simulink model "TP_MCA_QTP"  (R2025b)
settings: Solver=ode4  StartTime=0.0  StopTime=1000  FixedStep=1e-3  RelTol=1e-3
values from neighbouring files (symbols this model uses):
  A = full(A)    [Parameters.m]
  B = full(B)    [Parameters.m]
  QTP = {}    [Parameters.m]
  uref = sol(3:4)    [Parameters.m]
  xref = [href; sol(1:2)]    [Parameters.m]
undefined symbols (not defined in the file or in its folder): K
settings Model: Creator=yuqi  LastModifiedBy=flo

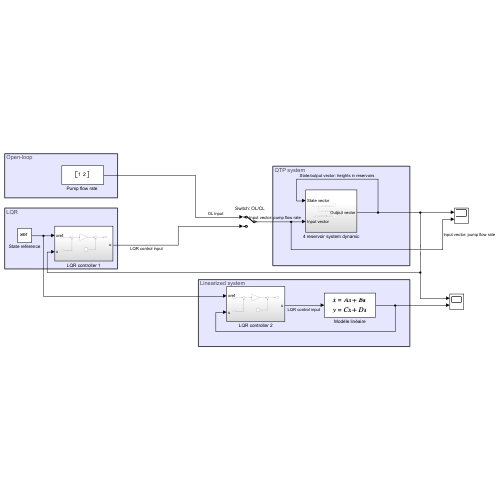
[thumbnail: Simulink's stored preview of the top-level diagram]
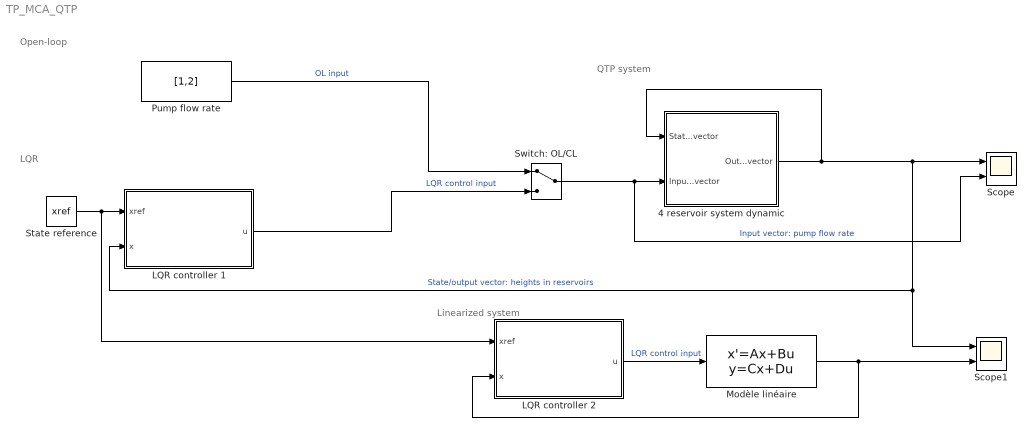
== system TP_MCA_QTP ==
  note: Linearized system
  note: Open-loop
  note: LQR
  note: QTP system
  4 reservoir system dynamic : Subsystem
  LQR controller 1 : Subsystem
  LQR controller 2 : Subsystem
  Modèle linéaire : StateSpace  A=A  B=B  C=eye(4)  D=zeros(4,2)  InitialCondition=QTP.h0
  "Pump flow rate " : Constant  Value=[1,2]
  Scope : Scope  NumInputPorts=2
      settings: ActiveDisplayYMinimum=-0.14202036556311504  ActiveDisplayYMaximum=1.3368369279989929
  Scope1 : Scope  NumInputPorts=2
      settings: ActiveDisplayYMinimum=-0.14887499999999998  ActiveDisplayYMaximum=1.349875
  State reference : Constant  Value=xref
  Switch: OL/CL : ManualSwitch
  wires:
  4 reservoir system dynamic/1(Output vector) -> Scope1/1, LQR controller 1/2(x), Scope/1, 4 reservoir system dynamic/1(State vector)  "State/output vector: heights in reservoirs"
  Switch: OL/CL/1 -> Scope/2, 4 reservoir system dynamic/2(Input vector)  "Input vector: pump flow rate"
  "Pump flow rate "/1 -> Switch: OL/CL/1  "OL input"
  State reference/1 -> LQR controller 2/1(xref), LQR controller 1/1(xref)
  LQR controller 1/1(u) -> Switch: OL/CL/2  "LQR control input"
  Modèle linéaire/1 -> LQR controller 2/2(x), Scope1/2
  LQR controller 2/1(u) -> Modèle linéaire/1  "LQR control input"

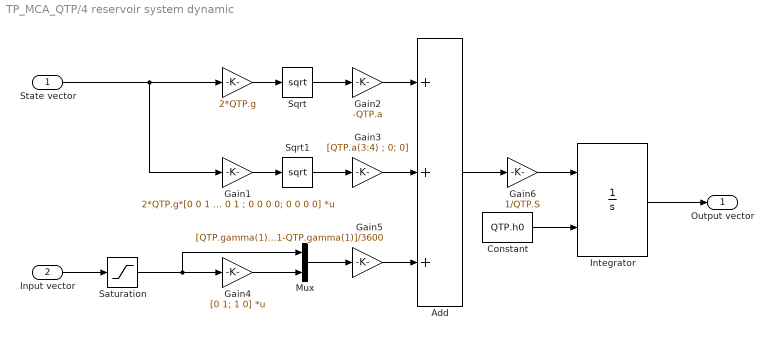
== system TP_MCA_QTP/4 reservoir system dynamic ==
  State vector : Inport
  Input vector : Inport  Port=2
  " " : Gain  Gain=2*QTP.g
  Add : Sum  Inputs=+++
  Constant : Constant  Value=QTP.h0
  Gain1 : Gain  Gain=2*QTP.g*[0 0 1 0; 0 0 0 1 ; 0 0 0 0; 0 0 0 0]  Multiplication=Matrix(K*u)
  Gain2 : Gain  Gain=-QTP.a
  Gain3 : Gain  Gain=[QTP.a(3:4) ; 0; 0]
  Gain4 : Gain  Gain=[0 1; 1 0]  Multiplication=Matrix(K*u)
  Gain5 : Gain  Gain=[QTP.gamma(1);QTP.gamma(2);1-QTP.gamma(2);1-QTP.gamma(1)]/3600
  Gain6 : Gain  Gain=1/QTP.S
  Integrator : Integrator  InitialConditionSource=external  LimitOutput=on  UpperSaturationLimit=QTP.hmax  LowerSaturationLimit=QTP.hmin
  Mux : Mux  Inputs=2
  Saturation : Saturate  UpperLimit=QTP.qmax  LowerLimit=QTP.qmin
  Sqrt : Sqrt
  Sqrt1 : Sqrt
  Output vector : Outport
  wires:
  Input vector/1 -> Saturation/1
  State vector/1 -> Gain1/1, " "/1
  Gain6/1 -> Integrator/1
  " "/1 -> Sqrt/1
  Gain1/1 -> Sqrt1/1
  Sqrt/1 -> Gain2/1
  Sqrt1/1 -> Gain3/1
  Gain2/1 -> Add/1
  Gain3/1 -> Add/2
  Gain4/1 -> Mux/2
  Mux/1 -> Gain5/1
  Gain5/1 -> Add/3
  Add/1 -> Gain6/1
  Integrator/1 -> Output vector/1
  Constant/1 -> Integrator/2
  Saturation/1 -> Mux/1, Gain4/1

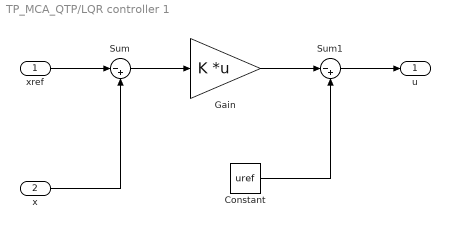
== system TP_MCA_QTP/LQR controller 1 ==
  xref : Inport
  x : Inport  Port=2
  Constant : Constant  Value=uref
  Gain : Gain  Gain=K  Multiplication=Matrix(K*u) (u vector)
  Sum : Sum  Inputs=|-+
  Sum1 : Sum  Inputs=|-+
  u : Outport
  wires:
  xref/1 -> Sum/1
  Sum/1 -> Gain/1
  x/1 -> Sum/2
  Gain/1 -> Sum1/1
  Sum1/1 -> u/1
  Constant/1 -> Sum1/2

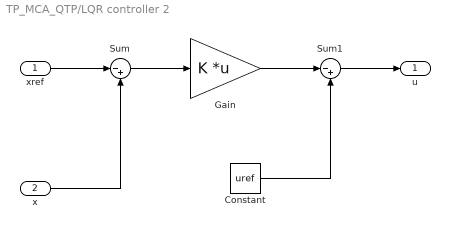
== system TP_MCA_QTP/LQR controller 2 ==
  xref : Inport
  x : Inport  Port=2
  Constant : Constant  Value=uref
  Gain : Gain  Gain=K  Multiplication=Matrix(K*u) (u vector)
  Sum : Sum  Inputs=|-+
  Sum1 : Sum  Inputs=|-+
  u : Outport
  wires:
  xref/1 -> Sum/1
  Sum/1 -> Gain/1
  x/1 -> Sum/2
  Gain/1 -> Sum1/1
  Sum1/1 -> u/1
  Constant/1 -> Sum1/2
